simulink model "Van_der_Pol"  (R2023b)
settings: Solver=VariableStepAuto  StartTime=0.0  StopTime=20.0  RelTol=1e-3
settings Model: Creator=mateisorodoc  LastModifiedBy=mateisorodoc

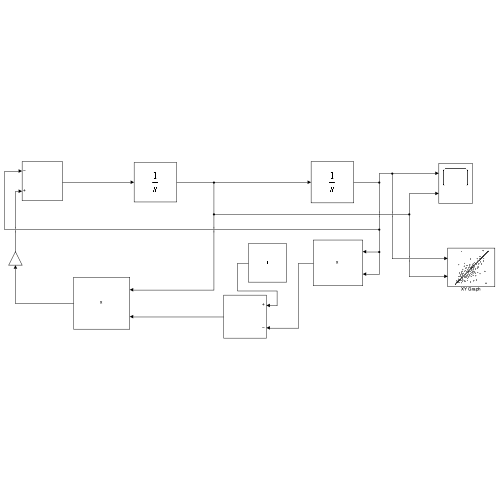
[thumbnail: Simulink's stored preview of the top-level diagram]
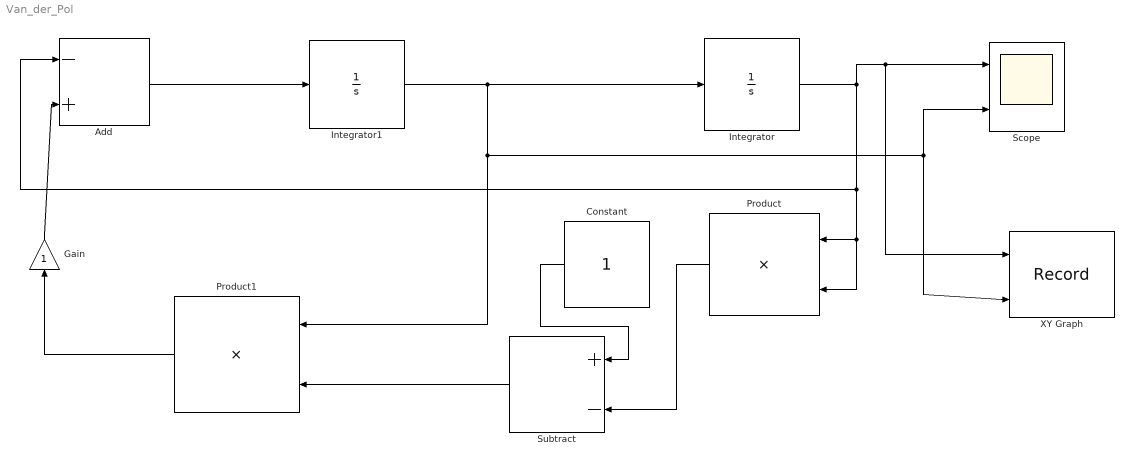
== system Van_der_Pol ==
  Add : Sum  Inputs=-+
  Constant : Constant
  Gain : Gain
  Integrator : Integrator  InitialCondition=0.5
  Integrator1 : Integrator  InitialCondition=-0.5
  Product : Product
  Product1 : Product
  Scope : Scope  NumInputPorts=2
  Subtract : Sum  Inputs=+-
  XY Graph : Record  FileSettingsInternal="{\"entries\":[{\"content\":{\"excelSettings\":{\"content\":{},\"type\":\"Streamout.ExcelSettings\"}},\"type\":\"Streamout.FileSettingStorage\",\"uuid\":\"\"}],\"packageUris\":[\"http:\\/\\/schema.mathworks.com\\/mf0\\/streamout_blocks\\/R2020a\"],\"version\":\"1.0\"}"  Layout=[1 1]  SignalsInternal="{\"entries\":[{\"content\":{\"signals\":[{\"content\":{\"blockPath\":[],\"dimensions\":[1],\"domain\":\"\",\"lineColor\":\"#a2142f\",\"plots\":[1],\"port\":1,\"sid\":[\"\"],\"signalID\":227,\"signalName\":\"Integrator\"},\"type\":\"RecordBlkView.Signal\",\"uuid\":\"\"},{\"content\":{\"blockPath\":[],\"dimensions\":[1],\"domain\":\"\",\"lineColor\":\"#139fff\",\"plots\":[1],\"port\":2,\"sid\":[\"\"],\"signalID\":231,\"signalName\":\"Integrator1\"},\"type\":\"RecordBlkView.Signal\",\"uuid\":\"\"}]},\"type\":\"RecordBlkView.InputSignals\",\"uuid\":\"\"}],\"packageUris\":[\"http:\\/\\/schema.mathworks.com\\/mf0\\/streamout_blocks\\/R2020a\"],\"version\":\"1.0\"}"  VisualizationBindings="{\"xyplotplugin\":{\"info\":[{\"series\":[{\"bindingParametersList\":[{\"parameter\":\"X-Axis\",\"signalID\":227,\"signalName\":\"Integrator\"},{\"parameter\":\"Y-Axis\",\"signalID\":231,\"signalName\":\"Integrator1\"}],\"seriesID\":31878}],\"subplotID\":1}]}}"  CompatibilityTag=XY  st=-1
  wires:
  Integrator/1 -> Product/2, Product/1, Add/1, XY Graph/1, Scope/1
  Product/1 -> Subtract/2
  Constant/1 -> Subtract/1
  Subtract/1 -> Product1/2
  Product1/1 -> Gain/1
  Add/1 -> Integrator1/1
  Gain/1 -> Add/2
  Integrator1/1 -> Scope/2, XY Graph/2, Product1/1, Integrator/1
